simulink model "FunctionalArchitectureProj"  (R2023b)
settings: Solver=VariableStepAuto  StartTime=0.0  StopTime=10.0  RelTol=1e-3
(part 3 of 3)

== system FunctionalArchitectureProj/Navigate the environment/Enable geofencing ==
  Bus Element In1 : Inport  PortName=position_accuracy
  Bus Element Out1 : Outport  PortName=geofencing_data

== system FunctionalArchitectureProj/Navigate the environment/Enable safe landing ==
  Bus Element In1 : Inport  PortName=stability_data
  Bus Element Out1 : Outport  PortName=Barometric_data

== system FunctionalArchitectureProj/Navigate the environment/Enhance position accuracy ==
  Bus Element In1 : Inport  PortName=position
  Bus Element Out1 : Outport  PortName=position_accuracy
  Bus Element Out2 : Outport  Port=2  PortName=accuracy-data

== system FunctionalArchitectureProj/Navigate the environment/Enhance stabilization  ==
  Bus Element In1 : Inport  PortName=orientation_feedback
  Bus Element Out1 : Outport  PortName=IMU_data

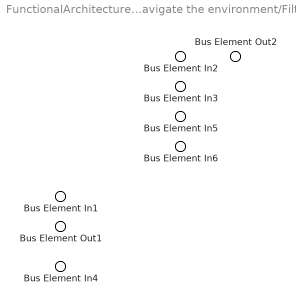
== system FunctionalArchitectureProj/Navigate the environment/Filtering ==
  Bus Element In5 : Inport  PortName=Airspeed
  Bus Element In6 : Inport  Port=2  PortName=Air_temperature
  Bus Element In3 : Inport  Port=3  PortName=IMU_data
  Bus Element In2 : Inport  Port=4  PortName=boundaries
  Bus Element In1 : Inport  Port=5  PortName=GNSS-data
  Bus Element In4 : Inport  Port=6  PortName=Barometric_data
  Bus Element Out2 : Outport  PortName=Drone_position
  Bus Element Out1 : Outport  Port=2  PortName=Drone_speed

== system FunctionalArchitectureProj/Navigate the environment/Improve flight stability ==
  Bus Element In1 : Inport  PortName=vertical_speed_data
  Bus Element Out1 : Outport  PortName=stability_data

== system FunctionalArchitectureProj/Navigate the environment/Improve performance in cold weather ==
  Bus Element In1 : Inport  PortName=changing_airspeed
  Bus Element Out1 : Outport  PortName=Airspeed
  Bus Element Out2 : Outport  Port=2  PortName=Air_temperature

== system FunctionalArchitectureProj/Navigate the environment/Localize boundaries ==
  Bus Element In1 : Inport  PortName=geofencing_data
  Bus Element Out1 : Outport  PortName=boundaries

== system FunctionalArchitectureProj/Navigate the environment/Measure airspeed ==
  Bus Element In1 : Inport  PortName=wind_data
  Bus Element Out1 : Outport  PortName=airspeed_data

== system FunctionalArchitectureProj/Navigate the environment/Measure angular velocity ==
  Bus Element In1 : Inport  PortName=Gyro_data
  Bus Element Out1 : Outport  PortName=velocity_data

== system FunctionalArchitectureProj/Navigate the environment/Measure atmospheric pressure ==
  Bus Element In2 : Inport  PortName=Power
  Bus Element In1 : Inport  Port=2  PortName=Environment_data
  Bus Element Out1 : Outport  PortName=altitude_data

== system FunctionalArchitectureProj/Navigate the environment/Measure orientation ==
  Bus Element In2 : Inport  PortName=Power
  Bus Element In1 : Inport  Port=2  PortName=Environment_data
  Bus Element Out1 : Outport  PortName=Gyro_data

== system FunctionalArchitectureProj/Navigate the environment/Monitor vertical speed ==
  Bus Element In1 : Inport  PortName=change_altitude
  Bus Element Out1 : Outport  PortName=vertical_speed_data

== system FunctionalArchitectureProj/Navigate the environment/Monitor wind speed ==
  Bus Element In2 : Inport  PortName=Power
  Bus Element In1 : Inport  Port=2  PortName=Environment_data
  Bus Element Out1 : Outport  PortName=wind_data

== system FunctionalArchitectureProj/Navigate the environment/Provide altitude data ==
  Bus Element In1 : Inport  PortName=altitude_data
  Bus Element Out1 : Outport  PortName=change_altitude

== system FunctionalArchitectureProj/Navigate the environment/Provide precise location ==
  Bus Element In2 : Inport  PortName=Power
  Bus Element In1 : Inport  Port=2  PortName=Environment_data
  Bus Element Out1 : Outport  PortName=position

== system FunctionalArchitectureProj/Navigate the environment/Support autopilot ==
  Bus Element In1 : Inport  PortName=airspeed_data
  Bus Element Out1 : Outport  PortName=critical_airspeed_data

== system FunctionalArchitectureProj/Navigate the environment/Track acceleration ==
  Bus Element In1 : Inport  PortName=velocity_data
  Bus Element Out1 : Outport  PortName=orientation_feedback

== system FunctionalArchitectureProj/Provide Energy/Charge battery ==
  Bus Element In1 : Inport  PortName=charging
  Bus Element Out1 : Outport  PortName=status

== system FunctionalArchitectureProj/Provide Energy/Manage the energy ==
  Bus Element In1 : Inport  PortName=Energy
  Bus Element Out2 : Outport  PortName=Power
  Bus Element Out1 : Outport  Port=2  PortName=charging

== system FunctionalArchitectureProj/Provide Energy/Monitor battery level ==
  Bus Element In1 : Inport  PortName=status

== system FunctionalArchitectureProj/Provide Energy/Provide energy  ==
  Bus Element In1 : Inport  PortName=BoxStationPower
  Bus Element Out1 : Outport  PortName=Energy

== system FunctionalArchitectureProj/Sense datas/Acquire images ==
  Bus Element In1 : Inport  PortName=Obstacles
  Bus Element In2 : Inport  Port=2  PortName=Power
  Bus Element Out1 : Outport  PortName=Camera_data
  Bus Element Out2 : Outport  Port=2  PortName=Camera_data1

== system FunctionalArchitectureProj/Sense datas/Analyze terrain ==
  Bus Element In1 : Inport  PortName=Landmarks_data
  Bus Element In2 : Inport  Port=2  PortName=lidar_data
  Bus Element Out1 : Outport  PortName=Terrain_data

== system FunctionalArchitectureProj/Sense datas/Detect objects ==
  Bus Element In1 : Inport  PortName=Camera_data
  Bus Element In2 : Inport  Port=2  PortName=Lidar_data
  Bus Element In3 : Inport  Port=3  PortName=ultrasonic_data
  Bus Element Out1 : Outport  PortName=Object_data

== system FunctionalArchitectureProj/Sense datas/Emit laser impulse ==
  Bus Element In1 : Inport  PortName=Obstacles
  Bus Element In2 : Inport  Port=2  PortName=Power
  Bus Element Out1 : Outport  PortName=laser_data

== system FunctionalArchitectureProj/Sense datas/Emit ultrasonic waves ==
  Bus Element In2 : Inport  PortName=Power
  Bus Element In1 : Inport  Port=2  PortName=Obstacles
  Bus Element Out1 : Outport  PortName=ultrasonic_data

== system FunctionalArchitectureProj/Sense datas/Filtering ==
  Bus Element In2 : Inport  PortName=Object_data
  Bus Element In1 : Inport  Port=2  PortName=Landing_data
  Bus Element Out1 : Outport  PortName=ObjectDetected

== system FunctionalArchitectureProj/Sense datas/Locate objects ==
  Bus Element In1 : Inport  PortName=Object_data
  Bus Element Out1 : Outport  PortName=Position_data

== system FunctionalArchitectureProj/Sense datas/Measure distance ==
  Bus Element In1 : Inport  PortName=speed_data
  Bus Element Out1 : Outport  PortName=ultrasonic_sensor_data

== system FunctionalArchitectureProj/Sense datas/Measure waves speed ==
  Bus Element In1 : Inport  PortName=waves
  Bus Element Out1 : Outport  PortName=speed_data

== system FunctionalArchitectureProj/Sense datas/Monitor delivery area ==
  Bus Element In1 : Inport  PortName=Terrain_data
  Bus Element Out1 : Outport  PortName=Landing_data

== system FunctionalArchitectureProj/Sense datas/Recognize landmarks ==
  Bus Element In1 : Inport  PortName=Camera_data1
  Bus Element Out1 : Outport  PortName=Landmarks_data

== system FunctionalArchitectureProj/Sense datas/Reflect impulse ==
  Bus Element In1 : Inport  PortName=laser_data
  Bus Element Out2 : Outport  PortName=Lidar_data
  Bus Element Out1 : Outport  Port=2  PortName=lidar_data

== system FunctionalArchitectureProj/Sense datas/Reflect waves ==
  Bus Element In1 : Inport  PortName=ultrasonic_data
  Bus Element Out1 : Outport  PortName=waves

== system FunctionalArchitectureProj/Sense datas/Track movements ==
  Bus Element In1 : Inport  PortName=Position_data
  Bus Element Out1 : Outport  PortName=Object_data

== system FunctionalArchitectureProj/Control the flight/Select mission step/Check mission state ==
  Bus Element In2 : Inport  PortName=Loaded Mission
  Bus Element In1 : Inport  Port=2  PortName=ActualPosition
  Bus Element Out2 : Outport  PortName=Mission Step

== system FunctionalArchitectureProj/Control the flight/Select mission step/Execute Cruise ==
  Bus Element In1 : Inport  PortName=Mission Step
  Bus Element Out1 : Outport  PortName=Cruise

== system FunctionalArchitectureProj/Control the flight/Select mission step/Execute Landing ==
  Bus Element In1 : Inport  PortName=Mission Step
  Bus Element Out1 : Outport  PortName=Landing

== system FunctionalArchitectureProj/Control the flight/Select mission step/Execute Take Off ==
  Bus Element In1 : Inport  PortName=Mission Step
  Bus Element Out1 : Outport  PortName=TakeOff

== system FunctionalArchitectureProj/Control the flight/Select mission step/Selected mission ==
  Bus Element In1 : Inport  PortName=TakeOff
  Bus Element In2 : Inport  Port=2  PortName=Cruise
  Bus Element In3 : Inport  Port=3  PortName=Landing
  Bus Element Out1 : Outport  PortName=Mission

== system FunctionalArchitectureProj/Deliver the payload/Detect door status/Ensure the status ==
  Bus Element In1 : Inport  PortName=Reed_data
  Bus Element Out1 : Outport  PortName=YES
  Bus Element Out2 : Outport  Port=2  PortName=NC
